simulink model "frft_qpsk_transceiver"  (R2025a)
settings: Solver=FixedStepDiscrete  StartTime=0.0  StopTime=1  RelTol=1e-3
PreLoadFcn:
  | % Add paths
  | addpath("dvb-s2/")
  | addpath("frft_filtering/")
  | addpath("gse")
  | 
  | 
  | 
  | 
  | setTxBurstLength = 10000;
  | txtmsg = ['Zynq radio HW/SW Co-design ÞÞÞÞ']; % Use only printable characters
  | 
  | %------------------------------------------------------------------------------------------------------
  | if ~isequal(size(txtmsg),[1 31])
  |     error('txtmsg must contain 31 characters');
  | end
  | 
  | [dataBits,msg] = zynqRadioHWSWQPSKgenHelloworldMsg(20); % generate 20 msgs for LUT
  | msgLUT = uint8(msg);
  | dataBitsLUT = dataBits(:);
  | Rsym                = 25e3;%1.92e6;
  | Config = zynqRadioHWSWQPSKTxRxParameters;
  | fs = Rsym*Config.SamplesPerSymbol;
  | word = [txtmsg newline];  % append a new line character to txtmsg
  | 
  | % The highest clock rate is 16 times the message character rate.
  | % As the message characters are fed at highest clock to FPGA
  | % repeat each character 16 times to maintain the message rate.
  | word = repelem(word.',16,1);
  | repeatTimes = ceil(setTxBurstLength/length(word));
  | inpData = complex(repmat(uint8(word),repeatTimes,1));
  | inUseTxBurstLength = length(inpData);
PostLoadFcn:
  | hScopeConfig = get_param([gcs '/HDL_QPSK/QPSK Tx Channel QPSK Rx/QPSK Rx/Frequency and Time Synchronizer/Symbol Synchronizer/No HDL/QPSK Receiver Eye Diagram'],'ScopeConfiguration');
  | hScopeConfig.OpenAtSimulationStart = false;
  | hScopeConfig.Visible = false;
  | clear hScopeConfig
InitFcn:
  | setTxBurstLength = 10000;
  | txtmsg = ['Zynq radio HW/SW Co-design ÞÞÞÞ']; % Use only printable characters
  | 
  | %------------------------------------------------------------------------------------------------------
  | if ~isequal(size(txtmsg),[1 31])
  |     error('txtmsg must contain 31 characters');
  | end
  | 
  | [dataBits,msg] = zynqRadioHWSWQPSKgenHelloworldMsg(20); % generate 20 msgs for LUT
  | msgLUT = uint8(msg);
  | dataBitsLUT = dataBits(:);
  | Rsym                = 25e3;%1.92e6;
  | Config = zynqRadioHWSWQPSKTxRxParameters;
  | fs = Rsym*Config.SamplesPerSymbol;
  | word = [txtmsg newline];  % append a new line character to txtmsg
  | 
  | % The highest clock rate is 16 times the message character rate.
  | % As the message characters are fed at highest clock to FPGA
  | % repeat each character 16 times to maintain the message rate.
  | word = repelem(word.',16,1);
  | repeatTimes = ceil(setTxBurstLength/length(word));
  | inpData = complex(repmat(uint8(word),repeatTimes,1));
  | inUseTxBurstLength = length(inpData);
undefined symbols (not defined in the file or in its folder): Add, dspblkCoreblockFVToolHelper, gcbh, Shift, unicode2native
libraries: hdlsllib x120, simulink x39, commseqgen3 x8, dsphdlsigops2 x4, whdledac x4, dsphdlfiltering2 x3, whdlutilities x3, dsphdlxfrm2 x2, dsphdlmathfun2 x2, commdigbbndpm3 x2, commchan3 x1, whdlmod x1
(part 4 of 5)

== system frft_qpsk_transceiver/Model Parameters/HDL_QPSK/QPSK Tx Channel QPSK Rx/QPSK Rx/Frequency and Time Synchronizer/Coarse Frequency Compensator/Raise Power to 4 ==
  dataIn : Inport
  validIn : Inport  Port=2
  Delay{1..8,11..12} (10 alike) : Delay
  Delay10 : Delay  DelayLength=1
  Delay9 : Delay  DelayLength=1
  Product1 : Product  OutDataTypeStr=Inherit: Same as first input
  Product2 : Product  OutDataTypeStr=Inherit: Same as first input
  dataOut : Outport
  validOut : Outport  Port=2
  wires:
  Delay12/1 -> validOut/1
  Delay11/1 -> dataOut/1
  Delay10/1 -> Delay8/1
  Delay9/1 -> Delay6/1, Delay7/1
  Delay8/1 -> Delay12/1
  Delay7/1 -> Product2/2
  Delay6/1 -> Product2/1
  Delay5/1 -> Delay2/1
  Delay4/1 -> Product1/2
  Delay3/1 -> Product1/1
  validIn/1 -> Delay5/1
  Product2/1 -> Delay11/1
  Delay2/1 -> Delay10/1
  Product1/1 -> Delay1/1
  Delay1/1 -> Delay9/1
  dataIn/1 -> Delay4/1, Delay3/1

== system frft_qpsk_transceiver/Model Parameters/HDL_QPSK/QPSK Tx Channel QPSK Rx/QPSK Rx/Frequency and Time Synchronizer/No HDL/Subsystem ==
  In1 : Inport
  Enable : EnablePort
  To Workspace : ToWorkspace  VariableName=simAfterCS  SampleTime=-1
      settings: Save2DSignal=2-D array (concatenate along first dimension)
  wires:
  In1/1 -> To Workspace/1

== system frft_qpsk_transceiver/Model Parameters/HDL_QPSK/QPSK Tx Channel QPSK Rx/QPSK Rx/Frequency and Time Synchronizer/PL Data Descrambler/PL Data Descrambler ==
  dataIn : Inport
  reset : Inport  Port=2
  validIn : Inport  Port=3
  Delay{2,4..5,7..8,10,22..23} (8 alike) : Delay  DelayLength=1
  Delay{15..17,20..21} (5 alike) : Delay
  Delay9 : Delay  DelayLength=7
  Math Function : Math  Operator=conj
  PL Scramble Sequence Mapper LUT : Lookup_n-D  NumberOfTableDimensions=1  LookupTableObject=''  BreakpointsSpecification=Even spacing  BreakpointsForDimension1=[-5:5]  BreakpointsForDimension1FirstPoint=0  BreakpointsForDimension2FirstPoint=10  BreakpointsForDimension2Spacing=12  IndexSearchMethod=Evenly spaced points  Table=[1;1i;-1;-1i]  TableDataTypeStr=fixdt(1,2,0)  InterpMethod=Flat  DiagnosticForOutOfRangeInput=Error  InternalRulePriority=Speed  OutDataTypeStr=fixdt(1,2,0)  RndMeth=Simplest
  PL Scrambler Gold Sequence Generator : Subsystem  mask{n=0}
      mask prompts: n "Index of Gold Sequence :"
  Product : Product  OutDataTypeStr=Inherit: Same as first input
  dataOut : Outport
  validOut : Outport  Port=2
  wires:
  PL Scrambler Gold Sequence Generator/1(dataOut) -> Delay2/1
  Math Function/1 -> Delay16/1
  dataIn/1 -> Delay9/1
  PL Scramble Sequence Mapper LUT/1 -> Delay7/1
  Product/1 -> Delay20/1
  PL Scrambler Gold Sequence Generator/2(validOut) -> Delay5/1
  reset/1 -> PL Scrambler Gold Sequence Generator/1(reset)
  validIn/1 -> PL Scrambler Gold Sequence Generator/2(validIn)
  Delay9/1 -> Delay4/1
  Delay2/1 -> PL Scramble Sequence Mapper LUT/1
  Delay4/1 -> Delay10/1
  Delay5/1 -> Delay8/1
  Delay7/1 -> Math Function/1
  Delay8/1 -> Delay17/1
  Delay10/1 -> Delay15/1
  Delay15/1 -> Product/1
  Delay16/1 -> Product/2
  Delay17/1 -> Delay21/1
  Delay21/1 -> Delay23/1
  Delay22/1 -> dataOut/1
  Delay23/1 -> validOut/1
  Delay20/1 -> Delay22/1

== system frft_qpsk_transceiver/Model Parameters/HDL_QPSK/QPSK Tx Channel QPSK Rx/QPSK Rx/Frequency and Time Synchronizer/Packet Controller/End Generator ==
  validIn : Inport
  rst : Inport  Port=2
  Compare To Constant : simulink/Logic and Bit Operations/Compare To Constant  relop===  const=size(cfg.frames,1)*8/2 -1  OutDataTypeStr=boolean
  Delay6 : Delay  DelayLength=1
  HDL Counter : hdlsllib/Sources/HDL Counter  CountType=Count limited  CountInit=0  CountStep=1  CountMax=size(cfg.frames,1)*8/2 -1  CountFromType=Initial value  CountFrom=0  CountResetPort=on  CountLoadPort=off  CountEnbPort=on  CountDirPort=off  CountHitOutputPort=off  CountDataType=Unsigned  CountWordLen=nextpow2(size(cfg.frames,1)*8/2 -1)  CountFracLen=0  CountSampTime=1
  Logical Operator1 : Logic  IconShape=distinctive  AllPortsSameDT=off  OutDataTypeStr=boolean
  endOut : Outport
  wires:
  Compare To Constant/1 -> Logical Operator1/1
  HDL Counter/1 -> Compare To Constant/1
  validIn/1 -> HDL Counter/2, Logical Operator1/2
  rst/1 -> HDL Counter/1
  Logical Operator1/1 -> Delay6/1
  Delay6/1 -> endOut/1

== system frft_qpsk_transceiver/Model Parameters/HDL_QPSK/QPSK Tx Channel QPSK Rx/QPSK Rx/Frequency and Time Synchronizer/Phase Ambiguity Estimation and Correction/Average Estimates ==
  endIn : Inport
  estin : Inport  Port=2
  validIn : Inport  Port=3
  Add : Sum  Inputs=++|
  Data Type Conversion : DataTypeConversion  OutDataTypeStr=fixdt(1,16+8,13)  SaturateOnIntegerOverflow=off  RndMeth=Floor
  Data Type Conversion1 : DataTypeConversion  OutDataTypeStr=fixdt(1,16+8,13)  SaturateOnIntegerOverflow=off  RndMeth=Floor
  Data Type Conversion2 : DataTypeConversion  OutDataTypeStr=fixdt(1,16,14)  SaturateOnIntegerOverflow=off  RndMeth=Floor
  Delay{,1..3} (4 alike) : Delay  DelayLength=1
  Divide by 8 : DataTypeConversion  OutDataTypeStr=fixdt(1,24,13+log2(8))  ConvertRealWorld=Stored Integer (SI)  SaturateOnIntegerOverflow=off  RndMeth=Floor
  Unit Delay Enabled Synchronous : hdlsllib/Discrete/Unit Delay Enabled Synchronous  InitialCondition=0.0  SampleTime=-1
  Unit Delay Enabled Resettable Synchronous : hdlsllib/Discrete/Unit Delay Enabled Resettable Synchronous  InitialCondition=0.0  SampleTime=-1
  avgEst : Outport
  wires:
  validIn/1 -> Delay1/1
  estin/1 -> Delay/1
  Data Type Conversion/1 -> Add/2
  Add/1 -> Data Type Conversion1/1
  Unit Delay Enabled Resettable Synchronous/1 -> Add/1, Divide by 8/1
  Data Type Conversion1/1 -> Unit Delay Enabled Resettable Synchronous/1
  Delay/1 -> Data Type Conversion/1
  Delay1/1 -> Unit Delay Enabled Resettable Synchronous/2
  endIn/1 -> Delay2/1
  Delay2/1 -> Delay3/1, Unit Delay Enabled Synchronous/2
  Delay3/1 -> Unit Delay Enabled Resettable Synchronous/3
  Divide by 8/1 -> Unit Delay Enabled Synchronous/1
  Unit Delay Enabled Synchronous/1 -> Data Type Conversion2/1
  Data Type Conversion2/1 -> avgEst/1

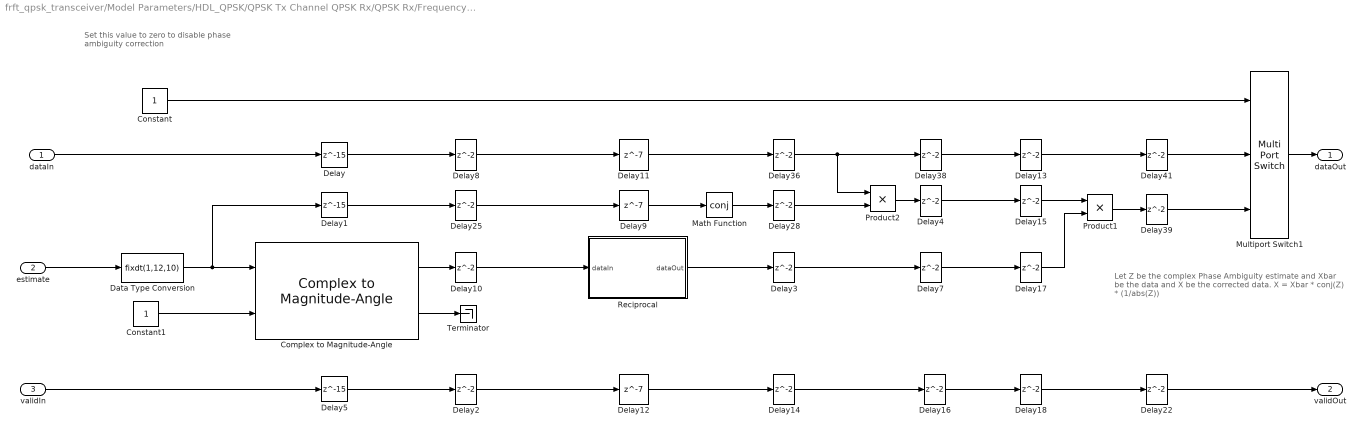
== system frft_qpsk_transceiver/Model Parameters/HDL_QPSK/QPSK Tx Channel QPSK Rx/QPSK Rx/Frequency and Time Synchronizer/Phase Ambiguity Estimation and Correction/Phase Ambiguity Corrector ==
  note: Let Z be the complex Phase Ambiguity estimate and Xbar be the data and X be the corrected data.
      | X = Xbar * conj(Z) * (1/abs(Z))
  note: Set this value to zero to disable phase ambiguity correction
  dataIn : Inport
  estimate : Inport  Port=2
  validIn : Inport  Port=3
  Complex to Magnitude-Angle : dsphdlmathfun2/Complex to Magnitude-Angle  NumIterationsSource=Auto  NumIterations=10  OutputFormat=Magnitude  AngleFormat=Normalized  ScaleOutput=on  ScalingMethod=Shift-Add  SimulateUsing=Code generation
  Constant : Constant  OutDataTypeStr=boolean  SampleTime=-1
  Constant1 : Constant  OutMin=1  OutMax=1  OutDataTypeStr=boolean  SampleTime=-1
  Data Type Conversion : DataTypeConversion  OutDataTypeStr=fixdt(1,12,10)  SaturateOnIntegerOverflow=off  RndMeth=Floor
  Delay : Delay  DelayLength=15
  Delay1 : Delay  DelayLength=15
  Delay{2..4,7..8,10,13..18,22,25,28,36,38..39,41} (19 alike) : Delay  InitialCondition=0
  Delay11 : Delay  DelayLength=7  InitialCondition=0
  Delay12 : Delay  DelayLength=7  InitialCondition=0
  Delay5 : Delay  DelayLength=15
  Delay9 : Delay  DelayLength=7  InitialCondition=0
  Math Function : Math  Operator=conj  SignedPower=on  RndMeth=Zero
  Multiport Switch1 : MultiPortSwitch  DataPortOrder=Zero-based contiguous  Inputs=2  zeroidx=on  SaturateOnIntegerOverflow=off  InputSameDT=off
  Product1 : Product  OutDataTypeStr=Inherit: Same as first input
  Product2 : Product  OutDataTypeStr=Inherit: Same as first input
  Reciprocal : Subsystem  mask{WL=13, FL=10, outWL=26, Mapp=RAM - Based}
      mask prompts: WL "Input Word Length :"; FL "Input Fractional Length :"; outWL "Output Word Length :"; Mapp "Mapping Type:"
      mask init:
      | % Inverse for 18 bit numbers: partitioned into 3+15 bits. 2^3 LUTs with 2^15
      | % combinations will store a total of 2^18 combinations.
      | % As each LUT has 2^15 combinations the data type of output has a maximum
      | % limit of 32 bits (2^20 is a maximum number of bits an LUT can store)
      | 
      | % Non tunable Parameters
      | % FL = 16;
      | % outWL = 31;
      | % WL = 18;
      | % This Parameter is not given for mask
      | LUTAddrWL = WL - 1; % this will implement 2 LUTs
      | 
      | % validate Non tunable parameters
      | % condition for validation: 2^20 bits is the maximum number of bits an LUT can store
      | if LUTAddrWL >= 20   % As 2^20 is the limit
      |     error('invalid LUTAddrWL');
      | end
      | if outWL >= 2^(20-LUTAddrWL)  % 2^(20-LUTAddrWL) is the maximum outWL based on condition for validation
      |     error('invalid outWL')
      | end
      | 
      | % calculate number of LUTs required
      | muxSelectorWL = WL - LUTAddrWL;
      | nLUT = 2^muxSelectorWL;
      | 
      | % Generate all possible RWV inputs using WL and FL
      | allInputRangeSI = -2^(WL-1):2^(WL-1)-1;  % as a stored integer
      | allInputRWV = allInputRangeSI * 2^(-FL);
      | 
      | % define the function for all the RWV input
      | reciprocal = 1./allInputRWV;
      | 
      | % store the function output in LUT
      | allLUTAddr = (0:2^LUTAddrWL-1);
      | LUT = zeros(length(allLUTAddr),nLUT);
      | for i = 0:nLUT-1
      |     LUT(:,i+1) = reciprocal(i*2^LUTAddrWL+1:(i+1)*2^LUTAddrWL);
      | end
      | 
      | % quantize the function with outWL
      | NT = numerictype(fi(LUT(abs(LUT) ~= inf),1,outWL)); % inf and -inf will be quantized with max and min values with NT data type
      | if NT.WordLength < NT. FractionLength
      |     NT.FractionLength = NT.WordLength
      | end
      | LUT = fi(LUT,NT);
      | 
      | paths = find_system([gcb '/Function Impl'],'BlockType','Delay');
      | 
      | for i = 1:length(paths)
      |     if Mapp == 1
      |         hdlset_param(paths{i},'ResetType','default');
      |     else
      |         hdlset_param(paths{i},'ResetType','none');
      |     end
      | end
      mask TypeOptions Mapp: LUT - Based | RAM - Based
      mask DialogControl DescGroupVar Prompt: LUT - Based function
      mask DialogControl DescTextVar Prompt: This block is implemented for complex reciprocal
      mask Display: disp(['Reciprocal\n' get_param(gcb,'Mapp') '\nLatency = 7'])
  Terminator : Terminator
  dataOut : Outport
  validOut : Outport  Port=2
  wires:
  Delay3/1 -> Delay7/1
  Delay18/1 -> Delay22/1
  Delay17/1 -> Product1/2
  Delay15/1 -> Product1/1
  Delay13/1 -> Delay41/1
  Delay10/1 -> Reciprocal/1(dataIn)
  Delay12/1 -> Delay14/1
  Delay11/1 -> Delay36/1
  Delay9/1 -> Math Function/1
  Delay4/1 -> Delay15/1
  Delay41/1 -> Multiport Switch1/2
  Delay8/1 -> Delay11/1
  Delay/1 -> Delay8/1
  dataIn/1 -> Delay/1
  validIn/1 -> Delay5/1
  Delay5/1 -> Delay2/1
  Delay2/1 -> Delay12/1
  Delay14/1 -> Delay16/1
  Product2/1 -> Delay4/1
  Multiport Switch1/1 -> dataOut/1
  Delay22/1 -> validOut/1
  Constant/1 -> Multiport Switch1/1
  Delay16/1 -> Delay18/1
  Delay28/1 -> Product2/2
  Math Function/1 -> Delay28/1
  Delay25/1 -> Delay9/1
  Delay1/1 -> Delay25/1
  Delay36/1 -> Product2/1, Delay38/1
  Delay38/1 -> Delay13/1
  estimate/1 -> Data Type Conversion/1
  Reciprocal/1(dataOut) -> Delay3/1
  Product1/1 -> Delay39/1
  Constant1/1 -> Complex to Magnitude-Angle/2
  Complex to Magnitude-Angle/1 -> Delay10/1
  Complex to Magnitude-Angle/2 -> Terminator/1
  Delay39/1 -> Multiport Switch1/3
  Delay7/1 -> Delay17/1
  Data Type Conversion/1 -> Delay1/1, Complex to Magnitude-Angle/1

== system frft_qpsk_transceiver/Model Parameters/HDL_QPSK/QPSK Tx Channel QPSK Rx/QPSK Rx/Frequency and Time Synchronizer/Phase Ambiguity Estimation and Correction/Phase Ambiguity Estimator ==
  dataIn : Inport
  syncPulse : Inport  Port=2
  validIn : Inport  Port=3
  Compare To Constant : simulink/Logic and Bit Operations/Compare To Constant  relop===  const=7  OutDataTypeStr=boolean
  Delay{1..3,8} (4 alike) : Delay  DelayLength=1
  Delay{4..7,9..11} (7 alike) : Delay
  Direct Lookup Table (n-D) : LookupNDDirect  NumberOfTableDimensions=1  Table=fi(preambleSymbols(3+1:3+8),1,16)  DiagnosticForOutOfRangeInput=Error
  HDL Counter : hdlsllib/Sources/HDL Counter  CountType=Count limited  CountInit=0  CountStep=1  CountMax=8-1  CountFromType=Initial value  CountFrom=0  CountResetPort=on  CountLoadPort=off  CountEnbPort=on  CountDirPort=off  CountHitOutputPort=off  CountDataType=Unsigned  CountWordLen=3  CountFracLen=0  CountSampTime=1
  Logical Operator : Logic  IconShape=distinctive  AllPortsSameDT=off  OutDataTypeStr=boolean
  Math Function : Math  Operator=conj  SignedPower=on  RndMeth=Zero
  Product : Product
  Subsystem : Subsystem
  Subsystem1 : Subsystem
  endOut : Outport
  estOut : Outport  Port=2
  validOut : Outport  Port=3
  wires:
  Compare To Constant/1 -> Logical Operator/2
  Subsystem/1(Out2) -> Subsystem1/1(In1), HDL Counter/1
  Direct Lookup Table (n-D)/1 -> Math Function/1
  Math Function/1 -> Delay4/1
  Product/1 -> Delay9/1
  Delay8/1 -> Direct Lookup Table (n-D)/1
  Delay1/1 -> Delay5/1
  Delay2/1 -> Delay6/1
  Delay3/1 -> Delay7/1
  Delay4/1 -> Product/2
  Delay5/1 -> Product/1
  Delay6/1 -> Delay10/1
  Delay7/1 -> Delay11/1
  Delay9/1 -> estOut/1
  Delay10/1 -> validOut/1
  Delay11/1 -> endOut/1
  dataIn/1 -> Delay1/1
  HDL Counter/1 -> Delay8/1, Compare To Constant/1
  Subsystem1/1(validOut) -> Delay2/1, Logical Operator/1, HDL Counter/2
  Logical Operator/1 -> Delay3/1, Subsystem/2(H)
  syncPulse/1 -> Subsystem/1(L)
  validIn/1 -> Subsystem1/2(validIn)

== system frft_qpsk_transceiver/Model Parameters/HDL_QPSK/QPSK Tx Channel QPSK Rx/QPSK Rx/Frequency and Time Synchronizer/Preamble Detector/Correlator ==
  dataIn : Inport
  validIn : Inport  Port=2
  Complex to Real-Imag : ComplexToRealImag  Output=Real
  Delay{1..6} (6 alike) : Delay  DelayLength=1
  Delay7 : Delay  DelayLength=4
  Delay8 : Delay  DelayLength=4
  Discrete FIR Filter : dsphdlfiltering2/Discrete FIR Filter  NumeratorSource=Property  Numerator=rxPreambleMFCoeffs  NumeratorPrototype=[]  FilterStructure=Direct form systolic  SerializationOption=Minimum number of cycles between valid input samples  NumCycles=2  NumberOfMultipliers=2  SimulateUsing=Code generation  roundingMode=Floor  overflowMode=off  CoefficientsDataTypeStr=Inherit: Same word length as input  OutputDataTypeStr=Inherit: Same word length as input  ResetInputPort=off  HDLGlobalReset=off  CoeffMultiplier=Multiplier  UseMultForPow2Coeff=on  FrameInputSymmOptim=off
  Magnitude Squared : Subsystem
  Magnitude Squared and Moving Sum : Subsystem
  ThresholdLimiter : MATLAB Function  TreatAsAtomicUnit=on
  dataOut : Outport
  threshold : Outport  Port=2
  validOut : Outport  Port=3
  wires:
  Discrete FIR Filter/2 -> Delay1/1
  validIn/1 -> Magnitude Squared and Moving Sum/2(validIn), Discrete FIR Filter/2
  Discrete FIR Filter/1 -> Delay6/1
  Delay1/1 -> Delay7/1
  Delay3/1 -> validOut/1
  dataIn/1 -> Magnitude Squared and Moving Sum/1(scaled1), Discrete FIR Filter/1
  Delay4/1 -> ThresholdLimiter/1(x)
  Delay2/1 -> dataOut/1
  Delay5/1 -> threshold/1
  Magnitude Squared and Moving Sum/1(E1) -> Delay4/1
  Delay6/1 -> Magnitude Squared/1(In1)
  Magnitude Squared/1(Out1) -> Complex to Real-Imag/1
  ThresholdLimiter/1(y) -> Delay8/1
  Delay7/1 -> Delay3/1
  Delay8/1 -> Delay5/1
  Complex to Real-Imag/1 -> Delay2/1

== system frft_qpsk_transceiver/Model Parameters/HDL_QPSK/QPSK Tx Channel QPSK Rx/QPSK Rx/Frequency and Time Synchronizer/Preamble Detector/No HDL ==
  In1 : Inport
  In2 : Inport  Port=2
  Enable : EnablePort
  Correlation Time Scope : Scope  NumInputPorts=2
      settings: TimeUnits=Metric (based on Time Span)  Title=Time Plot of Preamble Detection  ActiveDisplayYMinimum=-0.12629  ActiveDisplayYMaximum=1.13657  YLabel=Amplitude
  Data Type Conversion : DataTypeConversion  OutDataTypeStr=double  SaturateOnIntegerOverflow=off  RndMeth=Floor
  Data Type Conversion1 : DataTypeConversion  OutDataTypeStr=double  SaturateOnIntegerOverflow=off  RndMeth=Floor
  To Workspace : ToWorkspace  VariableName=simPeakFind  SampleTime=-1
      settings: Save2DSignal=2-D array (concatenate along first dimension)
  wires:
  Data Type Conversion1/1 -> Correlation Time Scope/2  "Threshold"
  In2/1 -> Data Type Conversion1/1
  Data Type Conversion/1 -> To Workspace/1, Correlation Time Scope/1  "Correlation Value"
  In1/1 -> Data Type Conversion/1

== system frft_qpsk_transceiver/Model Parameters/HDL_QPSK/QPSK Tx Channel QPSK Rx/QPSK Rx/Frequency and Time Synchronizer/Preamble Detector/Peak Search ==
  note: peak picker
  corr : Inport
  thresholdExceeded : Inport  Port=2
  validIn : Inport  Port=3
  Compare To Constant : simulink/Logic and Bit Operations/Compare To Constant  relop===  const=samplesPerFrame1x - 1  OutDataTypeStr=boolean
  Logical Operator : Logic  IconShape=distinctive  AllPortsSameDT=off  OutDataTypeStr=boolean
  Logical Operator4 : Logic  IconShape=distinctive  AllPortsSameDT=off  OutDataTypeStr=boolean
  Relational Operator : RelationalOperator  Operator=>  OutDataTypeStr=boolean  InputSameDT=off
  Terminator : Terminator
  Unit Delay Enabled Synchronous : hdlsllib/Discrete/Unit Delay Enabled Synchronous  InitialCondition=0.0  SampleTime=-1
  Unit Delay Enabled Synchronous1 : hdlsllib/Discrete/Unit Delay Enabled Synchronous  InitialCondition=0.0  SampleTime=-1
  Unit Delay Enabled Resettable Synchronous : hdlsllib/Discrete/Unit Delay Enabled Resettable Synchronous  InitialCondition=0.0  SampleTime=-1
  Unit Delay Enabled Resettable Synchronous1 : hdlsllib/Discrete/Unit Delay Enabled Resettable Synchronous  InitialCondition=0.0  SampleTime=-1
  timing Reference : hdlsllib/Sources/HDL Counter  CountType=Count limited  CountInit=0  CountStep=1  CountMax=samplesPerFrame1x - 1  CountFromType=Initial value  CountFrom=0  CountResetPort=off  CountLoadPort=off  CountEnbPort=on  CountDirPort=off  CountHitOutputPort=off  CountDataType=Unsigned  CountWordLen=nextpow2(samplesPerFrame1x - 1)  CountFracLen=0  CountSampTime=1
  timing Reference Long : hdlsllib/Sources/HDL Counter  CountType=Free running  CountInit=0  CountStep=1  CountMax=samplesPerFrame1x - 1  CountFromType=Initial value  CountFrom=0  CountResetPort=off  CountLoadPort=off  CountEnbPort=on  CountDirPort=off  CountHitOutputPort=off  CountDataType=Unsigned  CountWordLen=32  CountFracLen=0  CountSampTime=1
  timingOffset : Outport
  done : Outport  Port=2
  success : Outport  Port=3
  wires:
  validIn/1 -> Logical Operator/1, timing Reference/1, timing Reference Long/1
  timing Reference Long/1 -> Unit Delay Enabled Synchronous1/1
  timing Reference/1 -> Unit Delay Enabled Synchronous/1, Compare To Constant/1
  thresholdExceeded/1 -> Unit Delay Enabled Resettable Synchronous1/2, Unit Delay Enabled Resettable Synchronous1/1, Logical Operator4/2
  corr/1 -> Unit Delay Enabled Resettable Synchronous/1, Relational Operator/1
  Compare To Constant/1 -> Logical Operator/2
  Logical Operator/1 -> Unit Delay Enabled Resettable Synchronous1/3, done/1, Unit Delay Enabled Resettable Synchronous/3
  Relational Operator/1 -> Logical Operator4/1
  Unit Delay Enabled Resettable Synchronous/1 -> Relational Operator/2
  Unit Delay Enabled Resettable Synchronous1/1 -> success/1
  Logical Operator4/1 -> Unit Delay Enabled Synchronous/2, Unit Delay Enabled Synchronous1/2, Unit Delay Enabled Resettable Synchronous/2
  Unit Delay Enabled Synchronous/1 -> timingOffset/1
  Unit Delay Enabled Synchronous1/1 -> Terminator/1

== system frft_qpsk_transceiver/Model Parameters/HDL_QPSK/QPSK Tx Channel QPSK Rx/QPSK Rx/Frequency and Time Synchronizer/Preamble Detector/Timing Adjust ==
  timingOffset : Inport
  timingOffsetValid : Inport  Port=2
  dataIn : Inport  Port=3
  validIn : Inport  Port=4
  Delay{,1..4} (5 alike) : Delay  DelayLength=1
  Logical Operator : Logic  AllPortsSameDT=off  OutDataTypeStr=boolean
  Logical Operator1 : Logic  Operator=NOT  AllPortsSameDT=off  OutDataTypeStr=boolean
  Logical Operator2 : Logic  Inputs=3  AllPortsSameDT=off  OutDataTypeStr=boolean
  No HDL : Subsystem
  Relational Operator : RelationalOperator  Operator===  OutDataTypeStr=boolean  InputSameDT=off
  State Register : hdlsllib/Discrete/Unit Delay Enabled Resettable Synchronous  InitialCondition=0.0  SampleTime=-1
  Unit Delay Enabled Synchronous3 : hdlsllib/Discrete/Unit Delay Enabled Synchronous  InitialCondition=0.0  SampleTime=-1
  timing Reference : hdlsllib/Sources/HDL Counter  CountType=Count limited  CountInit=0  CountStep=1  CountMax=searchSamples - 1  CountFromType=Initial value  CountFrom=0  CountResetPort=off  CountLoadPort=off  CountEnbPort=on  CountDirPort=off  CountHitOutputPort=off  CountDataType=Unsigned  CountWordLen=nextpow2(searchSamples - 1)  CountFracLen=0  CountSampTime=1
  dataOut : Outport
  validOut : Outport  Port=2
  SyncPulse : Outport  Port=3
  wires:
  Delay4/1 -> dataOut/1
  Delay3/1 -> validOut/1
  timingOffset/1 -> Unit Delay Enabled Synchronous3/1
  Unit Delay Enabled Synchronous3/1 -> Relational Operator/2
  Delay/1 -> SyncPulse/1
  validIn/1 -> timing Reference/1, Logical Operator2/1, No HDL/1(validIn), Delay3/1
  State Register/1 -> Logical Operator2/3, Delay1/1
  Logical Operator1/1 -> Logical Operator/2
  Relational Operator/1 -> Logical Operator2/2
  Logical Operator2/1 -> No HDL/3(syncPulse), Delay/1, Delay2/1
  Delay2/1 -> State Register/3
  Logical Operator/1 -> State Register/1, State Register/2, Unit Delay Enabled Synchronous3/2
  timing Reference/1 -> No HDL/2(timingOffset), Relational Operator/1
  timingOffsetValid/1 -> Logical Operator/1
  Delay1/1 -> Logical Operator1/1
  dataIn/1 -> Delay4/1

== system frft_qpsk_transceiver/Model Parameters/HDL_QPSK/QPSK Tx Channel QPSK Rx/QPSK Rx/Frequency and Time Synchronizer/Symbol Synchronizer/Gardner TED ==
  data : Inport
  strobe : Inport  Port=2
  Constant : Constant  Value=0  OutDataTypeStr=Inherit: Inherit via back propagation  SampleTime=1/(Rsym*SamplesPerSymbol)
  Delay10 : Delay  DelayLength=4
  GTED : Subsystem
  Switch : Switch  Criteria=u2 ~= 0  InputSameDT=off
  e : Outport  VectorParamsAs1DForOutWhenUnconnected=off
  wires:
  Constant/1 -> Switch/3
  Switch/1 -> e/1
  strobe/1 -> Delay10/1
  data/1 -> GTED/1(In1)
  GTED/1(Out1) -> Switch/1
  Delay10/1 -> Switch/2

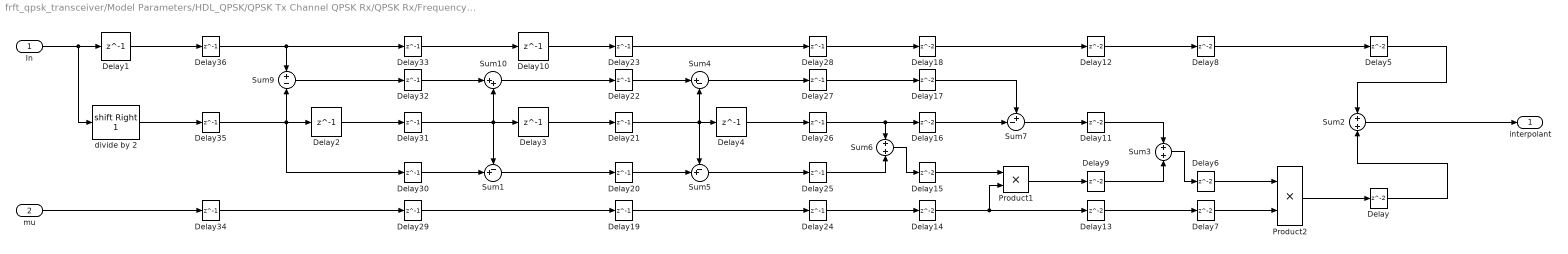
== system frft_qpsk_transceiver/Model Parameters/HDL_QPSK/QPSK Tx Channel QPSK Rx/QPSK Rx/Frequency and Time Synchronizer/Symbol Synchronizer/Interpolation Filter ==
  In : Inport
  mu : Inport  Port=2
  Delay{,5..9,11..18} (14 alike) : Delay
  Delay{1..4,10} (5 alike) : Delay  DelayLength=1  InitialCondition=0
  Delay{19..36} (18 alike) : Delay  DelayLength=1
  Product1 : Product  OutDataTypeStr=fixdt(1,16,10)  RndMeth=Zero
  Product2 : Product  RndMeth=Zero  OutDataTypeStr=Inherit: Same as first input
  Sum1 : Sum  Inputs=-+|
  Sum10 : Sum  Inputs=|++
  Sum2 : Sum  Inputs=+|+
  Sum3 : Sum  Inputs=+|+  OutDataTypeStr=fixdt(1,16,10)
  Sum4 : Sum  Inputs=|+-
  Sum5 : Sum  Inputs=-+|
  Sum6 : Sum  Inputs=+|+  OutDataTypeStr=fixdt(1,16,11)  SaturateOnIntegerOverflow=on
  Sum7 : Sum  Inputs=+-|  OutDataTypeStr=fixdt(1,16,10)
  Sum9 : Sum  Inputs=+-
  divide by 2 : ArithShift  BitShiftNumber=1  BitShiftDirection=Right
  interpolant : Outport
  wires:
  Sum9/1 -> Delay32/1
  In/1 -> divide by 2/1, Delay1/1
  Sum2/1 -> interpolant/1
  Sum7/1 -> Delay11/1
  Product1/1 -> Delay9/1
  Product2/1 -> Delay/1
  Sum3/1 -> Delay6/1
  Sum1/1 -> Delay20/1
  Delay3/1 -> Delay21/1
  Sum10/1 -> Delay22/1
  Delay2/1 -> Delay31/1
  Delay1/1 -> Delay36/1
  divide by 2/1 -> Delay35/1
  Delay/1 -> Sum2/2
  Delay5/1 -> Sum2/1
  Delay6/1 -> Product2/1
  Delay7/1 -> Product2/2
  Delay8/1 -> Delay5/1
  Delay9/1 -> Sum3/2
  Delay11/1 -> Sum3/1
  Delay12/1 -> Delay8/1
  Delay13/1 -> Delay7/1
  Delay14/1 -> Delay13/1, Product1/2
  Delay15/1 -> Product1/1
  Delay16/1 -> Sum7/2
  Delay17/1 -> Sum7/1
  Delay18/1 -> Delay12/1
  mu/1 -> Delay34/1
  Sum5/1 -> Delay25/1
  Delay4/1 -> Delay26/1
  Sum4/1 -> Delay27/1
  Delay10/1 -> Delay23/1
  Delay24/1 -> Delay14/1
  Sum6/1 -> Delay15/1
  Delay26/1 -> Delay16/1, Sum6/1
  Delay27/1 -> Delay17/1
  Delay28/1 -> Delay18/1
  Delay25/1 -> Sum6/2
  Delay19/1 -> Delay24/1
  Delay20/1 -> Sum5/2
  Delay21/1 -> Sum4/2, Sum5/1, Delay4/1
  Delay22/1 -> Sum4/1
  Delay23/1 -> Delay28/1
  Delay29/1 -> Delay19/1
  Delay30/1 -> Sum1/2
  Delay31/1 -> Sum1/1, Sum10/2, Delay3/1
  Delay32/1 -> Sum10/1
  Delay33/1 -> Delay10/1
  Delay34/1 -> Delay29/1
  Delay35/1 -> Delay30/1, Delay2/1, Sum9/2
  Delay36/1 -> Delay33/1, Sum9/1

== system frft_qpsk_transceiver/Model Parameters/HDL_QPSK/QPSK Tx Channel QPSK Rx/QPSK Rx/Frequency and Time Synchronizer/Symbol Synchronizer/Loop Filter ==
  note: Proportional-Plus-Integrator Loop Filter,
      | Infinite DC Response to guarantee convergence
  e : Inport
  Add : Sum
  Add2 : Sum  Inputs=|++  OutDataTypeStr=Inherit: Same as first input
  Data Type Conversion17 : DataTypeConversion  OutDataTypeStr=fixdt(1,11,10)  SaturateOnIntegerOverflow=off  RndMeth=Floor
  Delay : Delay  DelayLength=1
  Delay1 : Delay  DelayLength=1  InitialCondition=0
  Delay2 : Delay  InitialCondition=0
  Delay3 : Delay  InitialCondition=0
  Delay4 : Delay  DelayLength=1  InitialCondition=0
  Delay5 : Delay  InitialCondition=0
  Delay6 : Delay  DelayLength=1
  K1 : Gain  Gain=fi(SSLoopFilterPropGain,1,24,24)  ParamDataTypeStr=Inherit: Inherit from 'Gain'  OutDataTypeStr=fixdt(1,30,23)
  K2 : Gain  Gain=fi(SSLoopFilterIntegGain,1,24,24)  ParamDataTypeStr=Inherit: Inherit from 'Gain'  OutDataTypeStr=fixdt(1,30,23)
  v : Outport
  wires:
  Delay/1 -> Add2/2
  Delay5/1 -> Delay6/1
  Delay3/1 -> Delay1/1
  e/1 -> Delay2/1
  Add/1 -> Data Type Conversion17/1
  Delay1/1 -> Add/1
  Delay4/1 -> Add/2
  Delay2/1 -> K1/1, K2/1
  Data Type Conversion17/1 -> v/1
  K2/1 -> Delay5/1
  Add2/1 -> Delay/1, Delay4/1
  K1/1 -> Delay3/1
  Delay6/1 -> Add2/1

== system frft_qpsk_transceiver/Model Parameters/HDL_QPSK/QPSK Tx Channel QPSK Rx/QPSK Rx/Frequency and Time Synchronizer/Symbol Synchronizer/No HDL ==
  data : Inport
  valid : Inport  Port=2
  Data Type Conversion : DataTypeConversion  OutDataTypeStr=double  SaturateOnIntegerOverflow=off  RndMeth=Floor
  No HDL : Subsystem
  QPSK Receiver Eye Diagram : EyeDiagramBlock  WindowPosition=[177.000000,528.000000,1920.000000,977.000000,]  ScopeFrameLocation=window  SamplesPerSymbol=SamplesPerSymbol  SymbolsPerTrace=1  Title=RRC Matched Filtered Output  YLimits=[-1.1602,1.2629]
      settings: OpenAtSimulationStart=off
  Unit Delay Enabled Synchronous : hdlsllib/Discrete/Unit Delay Enabled Synchronous  InitialCondition=0.0  SampleTime=-1
  wires:
  data/1 -> No HDL/1(data), Unit Delay Enabled Synchronous/1
  Data Type Conversion/1 -> QPSK Receiver Eye Diagram/1
  Unit Delay Enabled Synchronous/1 -> Data Type Conversion/1
  valid/1 -> Unit Delay Enabled Synchronous/2, No HDL/Enable

== system frft_qpsk_transceiver/Model Parameters/HDL_QPSK/QPSK Tx Channel QPSK Rx/QPSK Rx/Frequency and Time Synchronizer/Symbol Synchronizer/Rate Handle ==
  dataIn : Inport
  strobe : Inport  Port=2
  validIn : Inport  Port=3
  Compare To Constant : simulink/Logic and Bit Operations/Compare To Constant  relop===  const=0  OutDataTypeStr=boolean
  Constant : Constant  Value=false  SampleTime=-1
  FIFO : Subsystem  mask{fifoSize=32*4, pushFullDiag=Error, popEmptyDiag=Ignore}
      mask prompts: fifoSize "FIFO size:"; pushFullDiag "Push full FIFO:"; popEmptyDiag "Pop empty FIFO:"
      mask TypeOptions pushFullDiag: Ignore | Warning | Error
      mask TypeOptions popEmptyDiag: Ignore | Warning | Error
  HDL Counter : hdlsllib/Sources/HDL Counter  CountType=Count limited  CountInit=0  CountStep=1  CountMax=SamplesPerSymbol - 1  CountFromType=Initial value  CountFrom=0  CountResetPort=off  CountLoadPort=off  CountEnbPort=on  CountDirPort=off  CountHitOutputPort=off  CountDataType=Unsigned  CountWordLen=nextpow2(SamplesPerSymbol - 1)  CountFracLen=0  CountSampTime=1
  Logical Operator : Logic  AllPortsSameDT=off  OutDataTypeStr=boolean
  Logical Operator1 : Logic  AllPortsSameDT=off  OutDataTypeStr=boolean
  Terminator : Terminator
  dataOut : Outport
  validOut : Outport  Port=2
  wires:
  dataIn/1 -> FIFO/1(in)
  validIn/1 -> Logical Operator1/2, Logical Operator/1, HDL Counter/1
  HDL Counter/1 -> Compare To Constant/1
  Compare To Constant/1 -> Logical Operator/2
  Logical Operator/1 -> FIFO/3(pop)
  FIFO/1(out) -> dataOut/1
  FIFO/3(validPop) -> validOut/1
  FIFO/2(numEntries) -> Terminator/1  "rx_fts_ss_rh_fifo_numEntries"
  Constant/1 -> FIFO/4(reset)
  strobe/1 -> Logical Operator1/1
  Logical Operator1/1 -> FIFO/2(push)

== system frft_qpsk_transceiver/Model Parameters/HDL_QPSK/QPSK Tx Channel QPSK Rx/QPSK Tx/Bit Packetizer/Data Bits FIFO/No HDL ==
  push : Inport
  pop : Inport  Port=2
  MATLAB Function : MATLAB Function  TreatAsAtomicUnit=on
  No HDL : Subsystem
  wires:
  push/1 -> MATLAB Function/1(wr), No HDL/1(push)
  pop/1 -> MATLAB Function/2(rd), No HDL/5(pop)
  MATLAB Function/2(ncount) -> No HDL/3(ncount)
  MATLAB Function/1(full) -> No HDL/2(full)
  MATLAB Function/3(empty) -> No HDL/4(empty)

== system frft_qpsk_transceiver/Model Parameters/HDL_QPSK/QPSK Tx Channel QPSK Rx/QPSK Tx/Bit Packetizer/Preamble Bits Generator/Preamble Bits Store ==
  note: The Preamble is padded with zeros in the LUT such that
      | the length is the 2^nextpow2(length(Preamble)) for
      | efficient resource mapping to RAM
  actualPreamble : Inport
  sampleCount : Inport  Port=2
  Constant : Constant  OutDataTypeStr=boolean  SampleTime=1/(Rsym*4)
  Extract Bits : simulink/Logic and Bit Operations/Extract Bits  bitsToExtract=Range of bits  numBits=8  bitIdxRange=[0 nextpow2(length(Preamble))-1]  outScalingMode=Treat bit field as an integer
  Preamble : LookupNDDirect  NumberOfTableDimensions=1  Table=[Preamble;false(32-length(Preamble),1)]  DiagnosticForOutOfRangeInput=Error
  Switch : Switch  Criteria=u2 ~= 0  Threshold=1  SaturateOnIntegerOverflow=off  InputSameDT=off
  preamble : Outport
  wires:
  Switch/1 -> preamble/1
  Constant/1 -> Switch/3
  Extract Bits/1 -> Preamble/1
  Preamble/1 -> Switch/1
  sampleCount/1 -> Extract Bits/1
  actualPreamble/1 -> Switch/2

== system frft_qpsk_transceiver/Model Parameters/HDL_QPSK/QPSK Tx Channel QPSK Rx/QPSK Tx/PL Data Scrambler/PL Scrambler Gold Sequence Generator/Subsystem ==
  note: The initial output of these outports are set to 0 as this is an enabled subsystem
  reset : Inport
  Enable : EnablePort
  X PN Generator M_n : commseqgen3/PN Sequence Generator  poly='z^18+z^7+1'  ini_sta=[zeros(1,17) 1]  outBitMaskSource=Dialog parameter  shift=n  outVarSiz=off  maxOutSizeMode=Dialog parameter  maxOutSize=[10 1]  Ts=-1  sampPerFrame=1  reset=on  bitPackedOutputs=off  outDataType=boolean  numPackedBits=8  bitPackDataSigned=off  bitPackedOutDType=double
  X PN Generator M_nplus131072 : commseqgen3/PN Sequence Generator  poly='z^18+z^7+1'  ini_sta=[zeros(1,17) 1]  outBitMaskSource=Dialog parameter  shift=n+131072  outVarSiz=off  maxOutSizeMode=Dialog parameter  maxOutSize=[10 1]  Ts=-1  sampPerFrame=1  reset=on  bitPackedOutputs=off  outDataType=boolean  numPackedBits=8  bitPackDataSigned=off  bitPackedOutDType=double
  Y PN Generator M_0 : commseqgen3/PN Sequence Generator  poly='z^18 + z^10 + z^7 + z^5 + 1'  ini_sta=ones(1,18)  outBitMaskSource=Dialog parameter  shift=0  outVarSiz=off  maxOutSizeMode=Dialog parameter  maxOutSize=[10 1]  Ts=-1  sampPerFrame=1  reset=on  bitPackedOutputs=off  outDataType=boolean  numPackedBits=8  bitPackDataSigned=off  bitPackedOutDType=double
  Y PN Generator M_131072 : commseqgen3/PN Sequence Generator  poly='z^18 + z^10 + z^7 + z^5 + 1'  ini_sta=ones(1,18)  outBitMaskSource=Dialog parameter  shift=131072  outVarSiz=off  maxOutSizeMode=Dialog parameter  maxOutSize=[10 1]  Ts=-1  sampPerFrame=1  reset=on  bitPackedOutputs=off  outDataType=boolean  numPackedBits=8  bitPackDataSigned=off  bitPackedOutDType=double
  xMnp131072 : Outport  InitialOutput=0
  yM131072 : Outport  Port=2  InitialOutput=0
  xMn : Outport  Port=3  InitialOutput=0
  yM0 : Outport  Port=4  InitialOutput=0
  wires:
  X PN Generator M_nplus131072/1 -> xMnp131072/1
  Y PN Generator M_0/1 -> yM0/1
  reset/1 -> X PN Generator M_nplus131072/1, Y PN Generator M_0/1, X PN Generator M_n/1, Y PN Generator M_131072/1
  X PN Generator M_n/1 -> xMn/1
  Y PN Generator M_131072/1 -> yM131072/1

== system frft_qpsk_transceiver/Model Parameters/HDL_QPSK/QPSK Tx Channel QPSK Rx/QPSK Rx/Frequency and Time Synchronizer/Coarse Frequency Compensator/Coarse Frequency Estimator/Extract Frequency ==
  datain : Inport
  validIn : Inport  Port=2
  Complex to Magnitude-Angle HDL Optimized : dsphdlmathfun2/Complex to Magnitude-Angle  NumIterationsSource=Auto  NumIterations=10  OutputFormat=Angle  AngleFormat=Normalized  ScaleOutput=on  ScalingMethod=Shift-Add  SimulateUsing=Code generation
  Delay{1..4} (4 alike) : Delay  DelayLength=1
  Gain : Gain  Gain=1/2  ParamDataTypeStr=fixdt(0,1,1)  OutDataTypeStr=Inherit: Same as input
  Unit Delay Enabled Synchronous : hdlsllib/Discrete/Unit Delay Enabled Synchronous  InitialCondition=0.0  SampleTime=-1
  normFreqOut : Outport
  wires:
  Unit Delay Enabled Synchronous/1 -> Delay2/1
  Complex to Magnitude-Angle HDL Optimized/2 -> Unit Delay Enabled Synchronous/2
  datain/1 -> Delay1/1
  Gain/1 -> Delay3/1
  Delay1/1 -> Complex to Magnitude-Angle HDL Optimized/1
  Delay2/1 -> Gain/1
  Delay3/1 -> normFreqOut/1
  validIn/1 -> Delay4/1
  Delay4/1 -> Complex to Magnitude-Angle HDL Optimized/2
  Complex to Magnitude-Angle HDL Optimized/1 -> Unit Delay Enabled Synchronous/1

== system frft_qpsk_transceiver/Model Parameters/HDL_QPSK/QPSK Tx Channel QPSK Rx/QPSK Rx/Frequency and Time Synchronizer/Coarse Frequency Compensator/Coarse Frequency Estimator/Integrator ==
  note: store the value in the Reg before reset
  dataIn : Inport
  validIn : Inport  Port=2
  Add1 : Sum  Inputs=|++  OutDataTypeStr=Inherit: Same as first input
  Delay : Delay  DelayLength=1
  Delay1 : Delay  DelayLength=1
  Delay2 : Delay  DelayLength=1
  Integ Reg : hdlsllib/Discrete/Unit Delay Enabled Resettable Synchronous  InitialCondition=0.0  SampleTime=-1
  Reset Generator : Subsystem
  Store Reg : hdlsllib/Discrete/Unit Delay Enabled Synchronous  InitialCondition=0.0  SampleTime=-1
  IntegOut : Outport
  IntegValid : Outport  Port=2
  wires:
  Add1/1 -> Integ Reg/1
  Integ Reg/1 -> Store Reg/1, Add1/2
  validIn/1 -> Delay2/1, Reset Generator/1(validIn)
  dataIn/1 -> Delay1/1
  Delay1/1 -> Add1/1
  Delay/1 -> IntegValid/1
  Store Reg/1 -> IntegOut/1
  Reset Generator/1(reset) -> Delay/1, Store Reg/2, Integ Reg/3
  Delay2/1 -> Integ Reg/2

== system frft_qpsk_transceiver/Model Parameters/HDL_QPSK/QPSK Tx Channel QPSK Rx/QPSK Rx/Frequency and Time Synchronizer/PL Data Descrambler/PL Data Descrambler/PL Scrambler Gold Sequence Generator ==
  reset : Inport
  validIn : Inport  Port=2
  Bit Concat : hdlsllib/Logic and Bit Operations/Bit Concat  numInputs=2
  Delay{,3..4,10,12..15} (8 alike) : Delay  DelayLength=1
  Delay{1..2,5..9,11} (8 alike) : Delay
  Logical Operator : Logic  Operator=XOR  AllPortsSameDT=off  OutDataTypeStr=boolean
  Logical Operator1 : Logic  Operator=XOR  AllPortsSameDT=off  OutDataTypeStr=boolean
  Logical Operator2 : Logic  Operator=OR  AllPortsSameDT=off  OutDataTypeStr=boolean
  Subsystem : Subsystem
  dataOut : Outport
  validOut : Outport  Port=2
  wires:
  Logical Operator2/1 -> Delay1/1
  Subsystem/4(yM0) -> Delay9/1
  Subsystem/3(xMn) -> Delay8/1
  Subsystem/2(yM131072) -> Delay7/1
  Subsystem/1(xMnp131072) -> Delay6/1
  reset/1 -> Delay3/1
  Bit Concat/1 -> Delay14/1
  Logical Operator/1 -> Delay12/1
  Logical Operator1/1 -> Delay10/1
  validIn/1 -> Delay4/1
  Delay/1 -> Delay11/1, Logical Operator2/2
  Delay11/1 -> Subsystem/1(reset)
  Delay1/1 -> Subsystem/Enable
  Delay2/1 -> Delay5/1
  Delay3/1 -> Delay/1
  Delay4/1 -> Logical Operator2/1, Delay2/1
  Delay5/1 -> Delay13/1
  Delay6/1 -> Logical Operator1/1
  Delay7/1 -> Logical Operator1/2
  Delay8/1 -> Logical Operator/1
  Delay9/1 -> Logical Operator/2
  Delay10/1 -> Bit Concat/1
  Delay12/1 -> Bit Concat/2
  Delay13/1 -> Delay15/1
  Delay14/1 -> dataOut/1
  Delay15/1 -> validOut/1

== system frft_qpsk_transceiver/Model Parameters/HDL_QPSK/QPSK Tx Channel QPSK Rx/QPSK Rx/Frequency and Time Synchronizer/Phase Ambiguity Estimation and Correction/Phase Ambiguity Corrector/Reciprocal ==
  dataIn : Inport
  Compare To Constant : simulink/Logic and Bit Operations/Compare To Constant  relop=<  const=0  OutDataTypeStr=boolean
  Data Type Conversion : DataTypeConversion  OutDataTypeStr=fixdt(1,WL,0)  ConvertRealWorld=Stored Integer (SI)  SaturateOnIntegerOverflow=off  RndMeth=Floor
  Data Type Conversion1 : DataTypeConversion  OutDataTypeStr=fixdt(0,LUTAddrWL,0)  ConvertRealWorld=Stored Integer (SI)  SaturateOnIntegerOverflow=off  RndMeth=Floor
  Data Type Conversion2 : DataTypeConversion  OutDataTypeStr=fixdt(0,WL-LUTAddrWL,0)  ConvertRealWorld=Stored Integer (SI)  SaturateOnIntegerOverflow=off  RndMeth=Floor
  Delay : Delay  DelayLength=1
  Delay1 : Delay  DelayLength=1
  Delay2 : Delay  DelayLength=1
  Extract Bits : simulink/Logic and Bit Operations/Extract Bits  bitsToExtract=Range ending with least significant bit  numBits=LUTAddrWL  bitIdxRange=[0 7]  outScalingMode=Treat bit field as an integer
  Function Impl : Subsystem
  dataOut : Outport
  wires:
  dataIn/1 -> Data Type Conversion/1
  Extract Bits/1 -> Delay2/1
  Data Type Conversion/1 -> Delay/1
  Compare To Constant/1 -> Delay1/1
  Data Type Conversion1/1 -> Function Impl/2(LUTAddr)
  Function Impl/1(functionValues) -> dataOut/1
  Delay/1 -> Compare To Constant/1, Extract Bits/1
  Delay1/1 -> Data Type Conversion2/1
  Delay2/1 -> Data Type Conversion1/1
  Data Type Conversion2/1 -> Function Impl/1(switch)

== system frft_qpsk_transceiver/Model Parameters/HDL_QPSK/QPSK Tx Channel QPSK Rx/QPSK Rx/Frequency and Time Synchronizer/Phase Ambiguity Estimation and Correction/Phase Ambiguity Estimator/Subsystem ==
  L : Inport
  H : Inport  Port=2
  Delay6 : Delay  DelayLength=1  InitialCondition=1
  Logical Operator : Logic  AllPortsSameDT=off  OutDataTypeStr=boolean
  Logical Operator1 : Logic  Operator=NOT  IconShape=distinctive  AllPortsSameDT=off  OutDataTypeStr=boolean
  Logical Operator2 : Logic  Operator=OR  AllPortsSameDT=off  OutDataTypeStr=boolean
  Out2 : Outport
  wires:
  L/1 -> Logical Operator1/1
  H/1 -> Logical Operator2/1
  Delay6/1 -> Out2/1, Logical Operator/2
  Logical Operator1/1 -> Logical Operator/1
  Logical Operator/1 -> Logical Operator2/2
  Logical Operator2/1 -> Delay6/1

== system frft_qpsk_transceiver/Model Parameters/HDL_QPSK/QPSK Tx Channel QPSK Rx/QPSK Rx/Frequency and Time Synchronizer/Phase Ambiguity Estimation and Correction/Phase Ambiguity Estimator/Subsystem1 ==
  In1 : Inport
  validIn : Inport  Port=2
  Logical Operator1 : Logic  IconShape=distinctive  AllPortsSameDT=off  OutDataTypeStr=boolean
  Logical Operator2 : Logic  Operator=NOT  IconShape=distinctive  AllPortsSameDT=off  OutDataTypeStr=boolean
  validOut : Outport
  wires:
  In1/1 -> Logical Operator2/1
  validIn/1 -> Logical Operator1/2
  Logical Operator1/1 -> validOut/1
  Logical Operator2/1 -> Logical Operator1/1

== system frft_qpsk_transceiver/Model Parameters/HDL_QPSK/QPSK Tx Channel QPSK Rx/QPSK Rx/Frequency and Time Synchronizer/Preamble Detector/Correlator/Magnitude Squared ==
  In1 : Inport
  Delay1 : Delay
  Delay2 : Delay
  Delay3 : Delay
  Math Function : Math  Operator=conj
  Product : Product
  Out1 : Outport
  wires:
  In1/1 -> Math Function/1, Delay2/1
  Math Function/1 -> Delay1/1
  Product/1 -> Delay3/1
  Delay2/1 -> Product/1
  Delay1/1 -> Product/2
  Delay3/1 -> Out1/1

== system frft_qpsk_transceiver/Model Parameters/HDL_QPSK/QPSK Tx Channel QPSK Rx/QPSK Rx/Frequency and Time Synchronizer/Preamble Detector/Correlator/Magnitude Squared and Moving Sum ==
  scaled1 : Inport
  validIn : Inport  Port=2
  Add : Sum  Inputs=|+-  OutDataTypeStr=Inherit: Same as first input
  Add1 : Sum  Inputs=|++  OutDataTypeStr=Inherit: Same as first input
  Complex to Real-Imag1 : ComplexToRealImag  Output=Real
  Delay : Delay  DelayLength=13  ShowEnablePort=on
      settings: InputPortMap=u0,e6
  Delay{1..4,6,8..10,12} (9 alike) : Delay
  Delay11 : Delay  DelayLength=11
  Delay14 : Delay  DelayLength=1  ShowEnablePort=on
      settings: InputPortMap=u0,e6
  Delay5 : Delay  DelayLength=1
  Delay7 : Delay  DelayLength=1
  Gain : Gain  Gain=ThresoldGainFac  OutDataTypeStr=Inherit: Same as input
  Math Function1 : Math  Operator=conj
  Product1 : Product
  E1 : Outport
  wires:
  Add/1 -> Delay5/1
  validIn/1 -> Delay12/1
  Delay/1 -> Add/2
  Delay14/1 -> Add1/2
  Complex to Real-Imag1/1 -> Delay3/1
  Add1/1 -> Delay11/1, Delay14/1
  Delay11/1 -> E1/1
  scaled1/1 -> Delay6/1, Math Function1/1
  Math Function1/1 -> Delay1/1
  Product1/1 -> Delay2/1
  Gain/1 -> Delay4/1
  Delay6/1 -> Product1/1
  Delay1/1 -> Product1/2
  Delay2/1 -> Complex to Real-Imag1/1
  Delay3/1 -> Gain/1
  Delay4/1 -> Delay/1, Add/1
  Delay5/1 -> Add1/1
  Delay7/1 -> Delay14/2
  Delay8/1 -> Delay/2, Delay7/1
  Delay9/1 -> Delay8/1
  Delay10/1 -> Delay9/1
  Delay12/1 -> Delay10/1

== system frft_qpsk_transceiver/Model Parameters/HDL_QPSK/QPSK Tx Channel QPSK Rx/QPSK Rx/Frequency and Time Synchronizer/Preamble Detector/Timing Adjust/No HDL ==
  note: This subsystem generates variables required for QPSKRxVerification for validation
  validIn : Inport
  timingOffset : Inport  Port=2
  syncPulse : Inport  Port=3
  Compare To Constant : simulink/Logic and Bit Operations/Compare To Constant  relop===  const=0  OutDataTypeStr=boolean
  Delay : Delay  DelayLength=4
  Delay1 : Delay  DelayLength=4
  Frame Counter : hdlsllib/Sources/HDL Counter  CountType=Free running  CountInit=0  CountStep=1  CountMax=bitsPerPacket/2 - 1  CountFromType=Initial value  CountFrom=0  CountResetPort=off  CountLoadPort=off  CountEnbPort=on  CountDirPort=off  CountHitOutputPort=off  CountDataType=Unsigned  CountWordLen=32  CountFracLen=0  CountSampTime=1
  Logical Operator : Logic  AllPortsSameDT=off  OutDataTypeStr=boolean
  No HDL : Subsystem
  No HDL1 : Subsystem
  Symbol Counter : hdlsllib/Sources/HDL Counter  CountType=Count limited  CountInit=0  CountStep=1  CountMax=bitsPerPacket/2 - 1  CountFromType=Initial value  CountFrom=0  CountResetPort=off  CountLoadPort=off  CountEnbPort=on  CountDirPort=off  CountHitOutputPort=off  CountDataType=Unsigned  CountWordLen=nextpow2(bitsPerPacket/2 - 1)  CountFracLen=0  CountSampTime=1
  Unit Delay Enabled Synchronous : hdlsllib/Discrete/Unit Delay Enabled Synchronous  InitialCondition=0.0  SampleTime=-1
  wires:
  timingOffset/1 -> Delay1/1
  validIn/1 -> Logical Operator/2, Symbol Counter/1
  Symbol Counter/1 -> Compare To Constant/1
  Logical Operator/1 -> Unit Delay Enabled Synchronous/2, Frame Counter/1
  Compare To Constant/1 -> Logical Operator/1
  Frame Counter/1 -> Unit Delay Enabled Synchronous/1
  syncPulse/1 -> Delay/1
  Unit Delay Enabled Synchronous/1 -> No HDL1/1(frameNumber)
  Delay/1 -> No HDL/Enable, No HDL1/Enable
  Delay1/1 -> No HDL/1(timingOffset)

== system frft_qpsk_transceiver/Model Parameters/HDL_QPSK/QPSK Tx Channel QPSK Rx/QPSK Rx/Frequency and Time Synchronizer/Symbol Synchronizer/Gardner TED/GTED ==
  In1 : Inport
  Add : Sum
  Add1 : Sum  Inputs=+-
  Add2 : Sum  Inputs=+-
  Complex to Real-Imag : ComplexToRealImag
  Delay{,1..7} (8 alike) : Delay  DelayLength=1
  Delay{8..13} (6 alike) : Delay
  Product : Product
  Product1 : Product
  Out1 : Outport
  wires:
  Product/1 -> Delay10/1
  Product1/1 -> Delay13/1
  Add/1 -> Out1/1
  In1/1 -> Complex to Real-Imag/1
  Complex to Real-Imag/1 -> Add1/2, Delay/1
  Delay3/1 -> Add1/1
  Delay/1 -> Delay1/1
  Delay2/1 -> Delay3/1
  Add1/1 -> Delay9/1
  Delay1/1 -> Delay2/1, Delay8/1
  Delay5/1 -> Delay11/1, Delay6/1
  Add2/1 -> Delay12/1
  Delay6/1 -> Delay7/1
  Delay4/1 -> Delay5/1
  Delay7/1 -> Add2/1
  Complex to Real-Imag/2 -> Add2/2, Delay4/1
  Delay8/1 -> Product/1
  Delay9/1 -> Product/2
  Delay10/1 -> Add/1
  Delay11/1 -> Product1/1
  Delay12/1 -> Product1/2
  Delay13/1 -> Add/2

== system frft_qpsk_transceiver/Model Parameters/HDL_QPSK/QPSK Tx Channel QPSK Rx/QPSK Rx/Frequency and Time Synchronizer/Symbol Synchronizer/No HDL/No HDL ==
  data : Inport
  Enable : EnablePort
  Data Type Conversion : DataTypeConversion  OutDataTypeStr=double  SaturateOnIntegerOverflow=off  RndMeth=Floor
  QPSK Receiver Constellation 1 : ConstellationDiagram  WindowPosition=[701.000000,587.000000,357.000000,388.000000,]  ScopeFrameLocation=window  SymbolsToDisplaySource=Property  SymbolsToDisplay=10000  Title=Before Symbol Synchronization  XLimits=[-1.9386 1.9401]  YLimits=[-1.9386 1.9401]  AxesLimits=[-1.9386 1.9401]  DefaultConfigurationName=comm.scopes.ConstellationDiagramBlockCfg
      settings: OpenAtSimulationStart=off
  To Workspace : ToWorkspace  VariableName=simBeforeSS  SampleTime=-1
      settings: Save2DSignal=2-D array (concatenate along first dimension)
  wires:
  Data Type Conversion/1 -> To Workspace/1, QPSK Receiver Constellation 1/1
  data/1 -> Data Type Conversion/1
